simulink model "dSpaceModel_2"  (R2023a)
settings: Solver=ode1  StartTime=0.0  StopTime=inf  FixedStep=0.001  RelTol=1e-3
PostLoadFcn:
  | , if any(exist('dsrtsu_mdlpostloadfcn', 'file') ~= 0), dsrtsu_mdlpostloadfcn('Execute', bdroot); end,
InitFcn:
  | , if any(exist('rtifpga_mdlclblib', 'file') ~= 0), rtifpga_mdlclblib('Init', bdroot); end,
model workspace (MAT data in the model file):
  mode = 2
libraries: rti1202serlib x5, simulink x2, svdutilitieslib x1
(part 3 of 3)

== stateflow chart dSpaceModel_2/RS485/THERMO FSM ==
  state IDLE [commented out]
    during:
    req_valid=false;
    if after(100, msec)
    req_valid=true;
    end
  state WAIT [commented out]
    entry:
    req_valid=false;
  state INIT
    % ZKDM replies are FC profile, fixed 8 bytes with BCC (XOR)
    str = "A005";
    addr = uint8('A005');
    expect_addr      = addr;      % uint8 (the on-wire address byte you use)
    expect_addr_len    = strlength(str);
    expect_len       = uint8(0);
    expect_crc_kind      = uint8(0);     % 0 = BCC/XOR
    % parser outputs (safe defaults)
    temp_rel    = 0.0;
    % Request interface defaults
    req_valid   = false;
    req_len     = uint8(0);
    %device
    last_ok_ms = uint32(0);
    comm_err_count = uint16(0);
  state READY
    entry:
    req_valid= false;
    READY_to_WAIT_GRANT = false;
    during:
    % Pacing: only build/send if enough time passed since last OK or last try
    if after(min_period_ms, msec)
    % Build the telegram NOW from live inputs
    [tx_buf, tx_len]  =  thermCom1(commandType, setpoint);
    %debug_pcd2 = tx_buf(1, 6:7);
    %debug_command = debug_cmnd(setpoint);
    % Advertise request to BUS MASTER
    req_bytes = tx_buf;
    req_len = tx_len;
    expect_addr  = addr;
    expect_len   = uint8(0);
    expect_crc_kind = uint8(0); % BCC XOR
    req_valid    = true;
    % move to wait for arbitration
    READY_to_WAIT_GRANT = true;
    end
  state COOLDOWN
    %nothing; the 'after(min_period_ms,msec)' in READY controls rate
  state HANDLE_ERR
    entry:
    comm_err_count = comm_err_count + 1;
    % Optionally: set FU_bereit=false when repeated timeouts
  state PARSE
    entry:
    temp_rel= parse_thermo_reply1(resp_data(1:64));
    % Master should have validated addr/len/BCC already; still allow a local guard:
    %if (bcc_ok)
    %tic();
    %last_ok_ms = uint32(toc());  % or leave; master’s timing is enough
    %else
    %comm_err_count = comm_err_count + uint16(1);
    %end
  state WAIT_RESP
    during:
    % keep req_valid_ZKDM = false to avoid re-queuing while current tx is active
    req_valid = false;
  state WAIT_GRANT
    %hold req_valid_ZKDM high until master grants
    entry:
    READY_to_WAIT_GRANT = false;
  (default) -> IDLE [commented out]
  WAIT -> IDLE [commented out] : [resp_ok || resp_err]
  IDLE -> WAIT [commented out] : [(after(1,tick))]
  (default) -> INIT
  COOLDOWN -> READY : [after(1,tick)]
  INIT -> READY : [(after(1,tick))]
  HANDLE_ERR -> COOLDOWN : [(after(1,tick))]
  PARSE -> COOLDOWN : after(min_period_ms,msec)
  WAIT_RESP -> HANDLE_ERR [order 2] : [resp_err>0]
  WAIT_GRANT -> HANDLE_ERR [order 2] : [resp_err>0]
  READY -> WAIT_GRANT : [    READY_to_WAIT_GRANT == true]
  WAIT_GRANT -> WAIT_RESP [order 1] : [grant==true]
  WAIT_RESP -> PARSE [order 1] : [resp_ok==true]
  data: address function_input; addressLength function_input; commandType function_input; setpoint function_input; setpointReduced function_input; setpointReducedLength function_input; command function_output; numBytes function_output; ctl_invalid function_input; run_en function_input; ref_pct function_input; bytes function_output; n function_output; commandType function_input; setpoint function_input; command function_output; length function_output; q14 function_input; pct function_output; commandType function_input; setpoint function_input; command function_output; outLen function_output; cfg function_output; buf function_input; n function_input; cfg function_input; ok function_output; status_word function_output uint16 size=1; freq_percent function_output; u function_input; y function_output; invalid_control_word function_input; active function_input; setpoint function_input; command function_output; off_set function_input; u function_input uint8 size=[1 64]; PCD1_1 function_output uint8 size=1; PCD1_2 function_output uint8 size=1; freq_rel_percent function_output double size=1; status_word function_output uint16 size=1; fu_ctrl_ready function_output boolean size=1; fu_ready function_output boolean size=1; fault_trip function_output boolean size=1; fault_no_trip function_output boolean size=1; bus_control_active function_output boolean size=1; bcc_ok function_output boolean size=1; setpoint function_input; cmnds function_output; pcd2 function_input; mode function_input; out function_output; b_in function_input; REV8 function_input; mode function_input; y function_output; REV8 function_output; active input boolean size=1; setpoint input double size=1; req_valid output boolean size=1; req_bytes output uint8 size=[1 127]; req_len output uint8 size=1; expect_addr output uint8; grant input boolean size=1; resp_ok input boolean size=1; resp_err input uint8 size=1; resp_data input uint8 size=[1 127]; resp_len input uint8 size=1; expect_len output uint8 size=1; expect_crc_kind output uint8 size=1; addr local uint8; invalid_flag local boolean size=1 =false; min_period_ms local uint8 size=1 =50; off_set local double size=1 =0; tx_len local uint8 size=1 =0; PCD1_1 local uint8 size=1; PCD1_2 local uint8 size=1; bus_ctrl_active local boolean size=1 =true; debug_command local uint16 size=[1 8]; debug_pcd2 local uint8 size=[1 2]; fault_no_trip local boolean size=1; fault_trip local boolean size=1; temp_rel local double size=1; fu_ctrl_ready local boolean size=1; fu_ready local boolean size=1; last_ok_ms local uint32 size=1; status_word local uint16 size=1; READY_to_WAIT_GRANT local; bcc_ok local boolean size=1; comm_err_count local uint16 size=1; tx_buf local uint8 size=[1 127]; commandType input uint8 size=1; str local string; expect_addr_len local double size=1
  function [command, numBytes] = thermoCommand(address, addressLength, commandType, setpoint, setpointReduced, setpointReducedLength):
    | function [command, numBytes] = thermoCommand(address, addressLength, commandType, setpoint, setpointReduced, setpointReducedLength)
    | 
    | % Initialize the command array and number of bytes
    | command  = zeros(1, 127, 'uint8');
    | numBytes = uint8(0);
    | 
    | % Insert the thermostat address into the command array
    | indexStart = 1;
    | indexEnd   = addressLength;
    | command(indexStart:indexEnd) = address(1:addressLength);
    | 
    | % Determine the command vector based on the provided command type (commandType)
    | switch commandType
    |     case 0
    |         commandVector = uint8('out_mode_05');  % Stop the thermostat
    |     case 1
    |         commandVector = uint8('out_sp_00');    % Set working temperature 'T'
    |     case 2
    |         commandVector = uint8('in_pv_00');     % Actual bath temperature
    |     case 3
    |         commandVector = uint8('in_pv_01');     % Current heat output (%)
    |     case 4
    |         commandVector = uint8('status');       % Status and error messages
    |     otherwise
    |         error('Invalid command: commandType must be in [0, 4].');
    | end
    | 
    | % Insert the command vector into the command array
    | commandLength = length(commandVector);
    | indexStart = indexEnd + 1;
    | indexEnd   = indexStart + commandLength - 1;
    | 
    | % Check for potential overflow
    | if indexEnd > length(command)
    |     error('Command array overflow: cannot add command.');
    | end
    | command(indexStart:indexEnd) = commandVector(1:commandLength);
    | 
    | % If `setpoint` is not NaN, append it to the command
    | if ~isnan(setpoint)
    |     % Insert a space (ASCII 32) between the command and the `setpoint`
    |     indexStart = indexEnd + 1;
    |     command(indexStart) = uint8(32); % Space character
    |     indexEnd = indexStart; % Update indexEnd to the newly added space
    | 
    |     % Depending on `commandType`, handle setpoint insertion differently
    |     if commandType == 0
    |         % For command type 0, transform setpoint to character
    |         command(indexEnd + 1) = uint8(setpoint + 48); % Convert number to corresponding ASCII character
    |         indexEnd = indexEnd + 1; % Move to the next index
    |     else
    |         % For other commands, use `setpointReduced`
    |         indexStart = indexEnd + 1;
    |         indexEnd   = indexStart + setpointReducedLength - 1;
    | 
    |         % Check for potential overflow
    |         if indexEnd > length(command)
    |             error('Command array overflow: cannot add setpointReduced.');
    |         end
    |         command(indexStart:indexEnd) = setpointReduced(1:setpointReducedLength);
    |     end
    | end
    | 
    | % Insert the end character (Carriage Return)
    | indexStart = indexEnd + 1;
    | command(indexStart) = uint8(13); % ASCII for Carriage Return
    | 
    | % Update numBytes to the total number of valid bytes filled in the command
    | numBytes = uint8(indexStart);
    | 
    | end
  function [bytes, n] = build_pcd8(ctl_invalid, run_en, ref_pct):
    | function [bytes, n] = build_pcd8(ctl_invalid, run_en, ref_pct)
    |     % Call your tested MATLAB Function (Create FC-Protocol Command 8-Bytes)
    |     % Or inline the builder. Must return [1x8 uint8] and n=8.
    |     n = unit8(8);
    |     [bytes, n] = FC_Command_8Bytes(ctl_invalid, run_en, ref_pct);
    | end
  function [command, length] = thermCom (commandType, setpoint):
    | function [command, length] = thermCom (commandType, setpoint)
    |     strr = 'A005';
    |     address = uint8(strr);
    |     addressLength = strlength(strr);
    |     tmp = sprintf('%.2f', setpoint);
    |     setpointReduced = uint8(tmp);
    |     setpointReducedLength = strlength(tmp);
    |     [command, length] = thermoCommand(address, addressLength, commandType, setpoint, setpointReduced, setpointReducedLength);
    | end
  function pct = q14_to_percent(q14):
    | function pct = q14_to_percent(q14)
    |     pct = 100.0 * double(q14) / 16384.0;
    | end
  function [command, outLen] = thermCom1(commandType, setpoint):
    | function [command, outLen] = thermCom1(commandType, setpoint)
    |     %#codegen
    |     
    |     address = uint8('A005_');
    |     addressLength = uint32(4);
    |     
    |     MAXSP = 16; % enough for "-999999.99"
    |     setpointReduced = zeros(1, MAXSP, 'uint8');
    |     setpointReducedLength = uint32(0);
    |     
    |     % ---- format setpoint to "%.2f" into fixed buffer ----
    |     x = double(setpoint);
    |     if isnan(x) || isinf(x)
    |         % "NaN" fallback
    |         setpointReduced(1:3) = uint8('NaN');
    |         setpointReducedLength = uint32(3);
    |     else
    |         % sign
    |         idx = uint32(1);
    |         if x < 0
    |             setpointReduced(idx) = uint8('-'); idx = idx + 1;
    |             x = -x;
    |         end
    |     
    |         % round to 2 decimals
    |         x100 = floor(x * 100 + 0.5);          % integer of value*100 rounded
    |         ip = floor(x100 / 100);               % integer part
    |         fp = x100 - ip * 100;                 % fractional part 0..99
    |     
    |         % integer part to ASCII (no leading zeros)
    |         % collect digits in reverse then write back
    |         tmpDigits = zeros(1, 10, 'uint8');
    |         dlen = uint32(0);
    |         if ip == 0
    |             dlen = uint32(1);
    |             tmpDigits(1) = uint8('0');
    |         else
    |             while ip > 0 && dlen < 10
    |                 dlen = dlen + 1;
    |                 digit = uint8(mod(ip,10));
    |                 tmpDigits(dlen) = uint8('0') + digit;
    |                 ip = floor(ip / 10);
    |             end
    |         end
    |         % write digits reversed
    |         for k = dlen:-1:1
    |             setpointReduced(idx) = tmpDigits(k);
    |             idx = idx + 1;
    |         end
    |     
    |         % decimal point
    |         setpointReduced(idx) = uint8('.'); idx = idx + 1;
    |     
    |         % two fractional digits (always)
    |         tens = uint8(floor(fp / 10));
    |         ones = uint8(fp - double(tens) * 10);
    |         setpointReduced(idx) = uint8('0') + tens; idx = idx + 1;
    |         setpointReduced(idx) = uint8('0') + ones; idx = idx + 1;
    |     
    |         setpointReducedLength = idx - 1;
    |     end
    |     
    |     [command, outLen] = thermoCommand( ...
    |         address, addressLength, commandType, setpoint, ...
    |         setpointReduced, setpointReducedLength);
    | end
  function cfg = zkdm_resp_map:
    | function cfg = zkdm_resp_map()
    | % Positions are 1-based indices in the received byte vector
    | cfg.idx_stx   = 1;
    | cfg.idx_len   = 2;
    | cfg.idx_addr  = 3;
    | cfg.idx_statH = 4;
    | cfg.idx_statL = 5;
    | cfg.idx_freqH = 6;
    | cfg.idx_freqL = 7;
    | cfg.idx_bcc   = 8;
    | 
    | cfg.expect_len = 8;        % total bytes
    | cfg.endian_hi_lo = true;   % Q14 is [HI, LO]
    | cfg.q14_fullscale = 16384; % 100%
    | end
  function [ok, status_word, freq_percent] = parse_fc_status(buf, n, cfg):
    | function [ok, status_word, freq_percent] = parse_fc_status(buf, n, cfg)
    | % buf: uint8 vector of the validated reply
    | % n  : actual length (== cfg.expect_len if master validated length)
    | % cfg: map from zkdm_resp_map()
    | 
    | ok = false;
    | status_word = uint16(0);
    | freq_percent = 0.0;
    | 
    | % Basic shape check (defensive)
    | if n < cfg.expect_len
    |     return;
    | end
    | 
    | % Status word (Bytes 4..5 by default)
    | stat_hi = uint16(buf(cfg.idx_statH));
    | stat_lo = uint16(buf(cfg.idx_statL));
    | status_word = bitor( stat_lo, bitshift(stat_hi, 8) );  % (HI,LO) → 16-bit
    | 
    | % Q14 output frequency (Bytes 6..7 by default)
    | bH = uint16(buf(cfg.idx_freqH));
    | bL = uint16(buf(cfg.idx_freqL));
    | if cfg.endian_hi_lo
    |     q14 = bitor( bL, bitshift(bH, 8) );     % HI,LO on the wire → H<<8 | L
    | else
    |     q14 = bitor( bH, bitshift(bL, 8) );     % LO,HI variant if needed
    | end
    | 
    | % Clip and scale to percent
    | if q14 > cfg.q14_fullscale
    |     q14 = cfg.q14_fullscale;   % sanity
    | end
    | freq_percent = 100.0 * double(q14) / double(cfg.q14_fullscale);
    | 
    | ok = true;
    | end
  function y = parse_thermo_reply1(u):
    | function y = parse_thermo_reply1(u)
    |     %#codegen
    |     % u: uint8 vector (e.g., 1x64)
    |     % returns y as double (NaN if invalid)
    |     
    |     y = NaN;
    |     
    |     N = int32(numel(u));
    |     if N == 0
    |         return;
    |     end
    |     
    |     CR = uint8(13);
    |     US = uint8('_');
    |     
    |     % ---------- find end (before CR) ----------
    |     endIdx = N;
    |     for i = int32(1):N
    |         if u(i) == CR
    |             endIdx = i - 1;
    |             break;
    |         end
    |     end
    |     if endIdx < 1
    |         return;
    |     end
    |     
    |     % ---------- find first underscore ----------
    |     sepIdx = int32(0);
    |     for i = int32(1):endIdx
    |         if u(i) == US
    |             sepIdx = i;
    |             break;
    |         end
    |     end
    |     if sepIdx == 0 || sepIdx == endIdx
    |         return;
    |     end
    |     
    |     % ---------- parse number after underscore ----------
    |     i = sepIdx + 1;
    |     
    |     % % skip spaces (optional)
    |     % while i <= endIdx && u(i) == uint8(32)
    |     %     i = i + 1;
    |     % end
    |     % if i > endIdx
    |     %     return;
    |     % end
    |     
    |     % sign
    |     sgn = 1.0;
    |     if u(i) == uint8('-')
    |         sgn = -1.0;
    |         i = i + 1;
    |     elseif u(i) == uint8('+')
    |         i = i + 1;
    |     end
    |     if i > endIdx
    |         return;
    |     end
    |     
    |     % integer part
    |     val = 0.0;
    |     hasDigit = false;
    |     while i <= endIdx
    |         c = u(i);
    |         if c >= uint8('0') && c <= uint8('9')
    |             val = val * 10.0 + double(c - uint8('0'));
    |             hasDigit = true;
    |             i = i + 1;
    |         else
    |             break;
    |         end
    |     end
    |     
    |     % fractional part
    |     if i <= endIdx && u(i) == uint8('.')
    |         i = i + 1;
    |         place = 0.1;
    |         while i <= endIdx
    |             c = u(i);
    |             if c >= uint8('0') && c <= uint8('9')
    |                 val = val + double(c - uint8('0')) * place;
    |                 place = place * 0.1;
    |                 hasDigit = true;
    |                 i = i + 1;
    |             else
    |                 break;
    |             end
    |         end
    |     end
    |     
    |     if ~hasDigit
    |         return;
    |     end
    |     
    |     y = sgn * val;
    | end
  function command = fcn(invalid_control_word, active, setpoint, off_set):
    | % Generates a telegram of the FC protocol for communication with a Danfoss frequency converter,
    | % telegram type: Process block (PCD) – 4 bytes
    | %
    | %##################################################################################
    | %Danfoss control word according to FC profile
    | %----------------------------------------------------------------------------------
    | %| Bit|                        Bit value = 0 |                     Bit value = 1  |
    | %|----|--------------------------------------|------------------------------------|
    | %| 00 | selection between the four "3-10 Preset reference [0]...[3]"             |
    | %| 01 | --""--                                                                   |
    | %|----|--------------------------------------|------------------------------------|
    | %| 02 |             DC brake and stop        |             performs ramp          |
    | %|----|--------------------------------------|------------------------------------|
    | %| 03 | lets the motor coast                 | starts the motor if conditions are met |
    | %|----|--------------------------------------|------------------------------------|
    | %| 04 | motor speed decreases until stop     |                                    |
    | %|----|--------------------------------------|------------------------------------|
    | %| 05 | current output frequency is stored   |                                    |
    | %|----|--------------------------------------|------------------------------------|
    | %| 06 | stop using ramp time                 | starts the motor if conditions are met |
    | %|----|--------------------------------------|------------------------------------|
    | %| 07 | no reset                             | reset                              |
    | %|----|--------------------------------------|------------------------------------|
    | %| 08 |                                      | output frequency "3-19 Jog [RPM]"  |
    | %|----|--------------------------------------|------------------------------------|
    | %| 09 | ramp 1 active ("3-41" and "3-42")    | ramp 2 active ("3-51" and "3-52")  |
    | %|----|--------------------------------------|------------------------------------|
    | %| 10 | control word is ignored              | control word is used               |
    | %|----|--------------------------------------|------------------------------------|
    | %| 11 | relay 01 not activated               | relay 01 activated                 |
    | %|----|--------------------------------------|------------------------------------|
    | %| 12 | relay 04 not activated               | relay 04 activated                 |
    | %|----|--------------------------------------|------------------------------------|
    | %| 13 | parameter set selection "0-10" and "8-55"                                |
    | %| 14 |                                                                            |
    | %|----|--------------------------------------|------------------------------------|
    | %| 15 | no reversal                          | reversal                           |
    | %----------------------------------------------------------------------------------
    | %##################################################################################
    | 
    | function command = fcn(invalid_control_word, active, setpoint, off_set)
    | 
    | if setpoint < 0
    |         error('setpoint must be non-negative.');
    | end
    | 
    | command = zeros(1, 127, 'uint8');
    | startzeichen = uint8(2);    % Start character (STX)
    | telegrammlaenge = uint8(6); % Specifies telegram length: 6 or 14 data bytes (data bytes + address byte + checksum)
    | adresse = 0b01111101;       % Address 125 in binary, address of the frequency converter (FU)
    |                             % Address format 1–126 => Bit 7 = 1; FU address “10” => Bit 0–6
    | pcd1_1 = 0b00000100;        % Control word (CTW) bits 15 to 08
    | pcd1_2 = 0b00100100;        % Control word (CTW) bits 07 to 00 ... before change: 0b00101110;
    | bcc = 0;                    % Data control byte, Block Check Character (BCC)
    | 
    | % modify the flag
    | if (invalid_control_word == false)
    |     pcd1_1 = bitor(pcd1_1, 0b00100000); 
    |     % If invalid_flag is `false`, the result will change `pcd11` to `0b00100000`, indicating that the control word is now in use.
    | end
    | 
    | if (active == true)
    |     pcd1_2 = bitor(pcd1_2, 0b01111100); % set 02, 03, 04, 05, 06 to 1
    |     pcd1_1 = bitor(pcd1_1, 0b00000100); % Starts the motor; "0": the frequency converter lets the motor coast
    | end
    | 
    | %%- `command(4) = pcd1_1;`
    |   % - Value: This byte is constructed based on the input conditions (`steuerwort_invalid` and `aktiv`).
    |   % - It starts with `0b00000000` (initial value) and may have bits set:
    |   %   - Bit 5 is set to 1 if `steuerwort_invalid` is false (valid control word).
    |   %   - Bit 4 is set to 1 if `aktiv` is true (start command).
    |   % - As a result, if `aktiv` is true, the value changes:
    |   %     - From: `0b00100000`
    |   %     - To:   `0b00110000` (decimal 48), indicating that the motor should start.
    | 
    | % scale the speed setpoint
    | % Example: convert 50% speed to 16-bit integer
    | % 50% = (16384 / 100 * 50) = 8192
    | % 8192 = 0b1000000000000000 (binary)
    | 
    | if (setpoint <= off_set)
    |     setpoint = 0;
    | else
    |     setpoint = setpoint - off_set;
    | end
    | 
    | soll = setpoint * (16384 / 100); 
    | pcd2 = typecast(int16(soll),'uint8');
    | % pcd2 = flip(pcd2);
    | 
    | %This is a 16-bit integer converted to two bytes that represents the desired speed (drehzahl_Sollwert) scaled to a proper range.
    |    %- The speed is scaled by multiplying the `drehzahl_Sollwert` by `(16384 / 100)`, allowing for a representation of the speed setting as a 16-bit integer.
    |    %- This is then converted from an `int16` to `uint8`, giving two bytes: `pcd2(1)` and `pcd2(2)`, with the bytes being flipped to match byte order expectations.
    | 
    | bcc = bitxor(startzeichen, telegrammlaenge);
    | bcc = bitxor(bcc, adresse);
    | bcc = bitxor(bcc, pcd1_1);
    | bcc = bitxor(bcc, pcd1_2);
    | bcc = bitxor(bcc, pcd2(1));
    | bcc = bitxor(bcc, pcd2(2));
    | 
    | command(1) = startzeichen;
    | command(2) = telegrammlaenge;
    | command(3) = adresse;
    | command(4) = pcd1_1; %This byte functions as part of the control command to the motor, determining how it should behave.
    | command(5) = pcd1_2; %This byte also forms part of the control command. It usually contains predefined flags or control commands as per the motor's specification.
    | command(6:7) = pcd2; %This part of the command specifies the desired speed for the motor. from the user sollwert.
    | command(8) = bcc;
    | 
    | %example message:
    | 
    | %Address: 118 Motor Activation Flag: True Target Speed: 89% BCC is valid
    | %2 6 118 48 46 56 246 162
  function [PCD1_1, PCD1_2, freq_rel_percent, ...:
    | function [PCD1_1, PCD1_2, freq_rel_percent, ...
    |           status_word, ...
    |           fu_ctrl_ready, fu_ready, fault_trip, fault_no_trip, bus_control_active, ...
    |           bcc_ok] = parse_fc_reply(u)
    | %#codegen
    | % Parse 8-byte FC reply built by your current build_fc_rx_telegram()
    | % Layout: [STX, LEN, ADDR, STW_HI, STW_LO, OUT_HI, OUT_LO, BCC]
    | % Bit mapping (matches your TX builder with msbpos()):
    | %   fu_ctrl_ready      -> bit15
    | %   fu_ready           -> bit14
    | %   fault_trip         -> bit13
    | %   fault_no_trip      -> bit12
    | %   bus_control_active -> bit6
    | 
    |     % ---- basic checks ----
    |     if numel(u) < 8
    |         error('parse_fc_reply:BadLength','u must have at least 8 bytes');
    |     end
    |     u = uint8(u(:).'); % row uint8
    | 
    |     % ---- BCC (XOR of bytes 1..7) ----
    |     b = uint8(0);
    |     for k = 1:7
    |         b = bitxor(b, u(k));
    |     end
    |     bcc_ok = (b == u(8));
    | 
    |     % ---- status word bytes ----
    |     PCD1_1 = u(4); % high byte (bits 15..8)
    |     PCD1_2 = u(5); % low  byte (bits 7..0)
    | 
    |     % Full 16-bit status word: [HI<<8 | LO]
    |     status_word = bitor( bitshift(uint16(PCD1_1),8), uint16(PCD1_2) );
    | 
    |     % Helper to read a single LSB-indexed bit (0..15)
    |     getbit = @(w, n) bitand(w, bitshift(uint16(1), n)) ~= 0;
    | 
    |     % ---- flags (LSB indexing) matching your TX mapping ----
    |     fu_ctrl_ready      = getbit(status_word, 15); % msbpos(0)
    |     fu_ready           = getbit(status_word, 14); % msbpos(1)
    |     fault_trip         = getbit(status_word, 13); % msbpos(2)
    |     fault_no_trip      = getbit(status_word, 12); % msbpos(3)
    |     bus_control_active = getbit(status_word,  6); % msbpos(9)
    | 
    |     % ---- OUT (Q14) -> relative frequency (%) ----
    |     q14 = bitor( bitshift(uint16(u(6)),8), uint16(u(7)) );
    |     freq_rel_percent = double(q14) * (100.0/16384.0);
    | end
  function cmnds = debug_cmnd(setpoint):
    | function cmnds = debug_cmnd(setpoint)
    |     
    |     if setpoint < 0
    |             error('setpoint must be non-negative.');
    |     end
    |     
    |     command = zeros(1, 8, 'uint16');
    |     soll = setpoint * (16384 / 100); 
    |     pcd2 = uint16(round(soll));
    |     all = pcd2_flipcases(pcd2);
    |     cmnds = all.values;
    | end
  function out = pcd2_flipcases(pcd2, mode):
    | function out = pcd2_flipcases(pcd2, mode)
    | % Modes (YOUR numbering):
    | %   0: I
    | %   1: N
    | %   2: R    (per-byte bit reverse)
    | %   3: B    (byte swap)
    | %   4: BR   (byte swap + per-byte bit reverse)
    | %   5: NR
    | %   6: NB
    | %   7: NBR
    | 
    |     x = uint16(pcd2);
    |     origSize = size(x);
    |     x = x(:);
    | 
    |     b = reshape(typecast(x, 'uint8'), 2, []).';  % N-by-2 uint8, [LSB MSB]
    | 
    |     persistent REV8
    |     if isempty(REV8)
    |         REV8 = make_rev8_lut();
    |     end
    | 
    |     % Internal bitmask encoding (N=1, B=2, R=4) is convenient,
    |     % but you want a different external mode order:
    |     % external_mode -> internal_mask
    |     map = uint8([0 1 4 2 6 5 3 7]);
    | 
    |     labels = {"I","N","R","B","BR","NR","NB","NBR"};
    | 
    |     if nargin < 2 || isempty(mode)
    |         vals = zeros(numel(x), 8, 'uint16');
    |         for m = 0:7
    |             vals(:, m+1) = apply_mode(b, REV8, map(m+1));
    |         end
    |         out = struct();
    |         out.modes  = uint8(0:7);
    |         out.labels = labels;
    |         out.values = vals;                          % (numel(x) x 8)
    |         out.asArray = reshape(vals, [origSize, 8]); % append dim=8
    |         return;
    |     end
    | 
    |     mode = uint8(mode);
    |     if any(mode > 7)
    |         error("mode must be an integer in 0..7.");
    |     end
    | 
    |     if isscalar(mode)
    |         y = apply_mode(b, REV8, map(mode+1));
    |         out = reshape(y, origSize);
    |         return;
    |     end
    | 
    |     mode = mode(:).';
    |     vals = zeros(numel(x), numel(mode), 'uint16');
    |     for k = 1:numel(mode)
    |         vals(:, k) = apply_mode(b, REV8, map(mode(k)+1));
    |     end
    |     out = reshape(vals, [origSize, numel(mode)]);
    | end
  function y = apply_mode(b_in, REV8, mode):
    | function y = apply_mode(b_in, REV8, mode)
    |     % b_in: N-by-2 uint8, [LSB MSB]
    |     b = b_in;
    | 
    |     doN = bitand(mode, 1) ~= 0;
    |     doB = bitand(mode, 2) ~= 0;
    |     doR = bitand(mode, 4) ~= 0;
    | 
    |     if doN
    |         b = bitcmp(b);
    |     end
    | 
    |     if doR
    |         % per-byte bit reverse via LUT
    |         b = REV8(double(b) + 1);
    |     end
    | 
    |     if doB
    |         b = b(:, [2 1]); % swap bytes
    |     end
    | 
    |     % Back to uint16 (bytes must be laid out as [LSB MSB] for typecast)
    |     bb = b.';                        % 2-by-N
    |     y  = typecast(bb(:), 'uint16');  % N-by-1 uint16
    | end
  function REV8 = make_rev8_lut:
    | 
    | % function LUT = make_rev8_lut()
    | %     % Pure bit-ops LUT: LUT(v+1) = bit-reverse of uint8(v)
    | %     LUT = zeros(256, 1, 'uint8');
    | %     for v = 0:255
    | %         x = uint8(v);
    | %         r = uint8(0);
    | %         % reverse 8 bits
    | %         for k = 0:7
    | %             r = bitor(r, bitshift(bitand(x, bitshift(uint8(1), k)), 7-k) ~= 0);
    | %         end
    | %         LUT(v+1) = r;
    | %     end
    | % end
    | 
    | function REV8 = make_rev8_lut()
    |     %REV8(i) = bit-reversal of uint8(i-1)
    |     
    |     x = uint8(0:255);
    |     REV8 = zeros(1,256,'uint8');
    |     
    |     for i = 1:256
    |         b = x(i);
    |         r = uint8(0);
    |         for k = 0:7
    |             % bitget returns double -> cast to uint8 before shifting
    |             r = bitor(r, bitshift(uint8(bitget(b, k+1)), 7-k));
    |         end
    |         REV8(i) = r;
    |     end
    | end

== matlab function dSpaceModel_2/RS485/MATLAB Function2 ==
  data: u input; PCD1_1 output; PCD1_2 output; freq_rel_percent output; status_word output; fu_ctrl_ready output; fu_ready output; fault_trip output; fault_no_trip output; bus_control_active output; bcc_ok output
function [PCD1_1, PCD1_2, freq_rel_percent, ...
          status_word, ...
          fu_ctrl_ready, fu_ready, fault_trip, fault_no_trip, bus_control_active, ...
          bcc_ok] = parse_fc_reply(u)
%#codegen
% Parse 8-byte FC reply built by your current build_fc_rx_telegram()
% Layout: [STX, LEN, ADDR, STW_HI, STW_LO, OUT_HI, OUT_LO, BCC]
% Bit mapping (matches your TX builder with msbpos()):
%   fu_ctrl_ready      -> bit15
%   fu_ready           -> bit14
%   fault_trip         -> bit13
%   fault_no_trip      -> bit12
%   bus_control_active -> bit6

    % ---- basic checks ----
    if numel(u) < 8
        error('parse_fc_reply:BadLength','u must have at least 8 bytes');
    end
    u = uint8(u(:).'); % row uint8

    % ---- BCC (XOR of bytes 1..7) ----
    b = uint8(0);
    for k = 1:7
        b = bitxor(b, u(k));
    end
    bcc_ok = (b == u(8));

    % ---- status word bytes ----
    PCD1_1 = u(4); % high byte (bits 15..8)
    PCD1_2 = u(5); % low  byte (bits 7..0)

    % Full 16-bit status word: [HI<<8 | LO]
    status_word = bitor( bitshift(uint16(PCD1_1),8), uint16(PCD1_2) );

    % Helper to read a single LSB-indexed bit (0..15)
    getbit = @(w, n) bitand(w, bitshift(uint16(1), n)) ~= 0;

    % ---- flags (LSB indexing) matching your TX mapping ----
    fu_ctrl_ready      = getbit(status_word, 15); % msbpos(0)
    fu_ready           = getbit(status_word, 14); % msbpos(1)
    fault_trip         = getbit(status_word, 13); % msbpos(2)
    fault_no_trip      = getbit(status_word, 12); % msbpos(3)
    bus_control_active = getbit(status_word,  6); % msbpos(9)

    % ---- OUT (Q14) -> relative frequency (%) ----
    q14 = bitor( bitshift(uint16(u(6)),8), uint16(u(7)) );
    freq_rel_percent = double(q14) * (100.0/16384.0);
end

== matlab function dSpaceModel_2/RS485/Subsystem2/MATLAB Function ==
  data: u input; PCD1_1 output; PCD1_2 output; PCD2 output
function [PCD1_1, PCD1_2, PCD2] = fcn(u)
%Steuerwort
PCD1_1 = u(4);
PCD1_2 = u(5);

%berechnet aktuelle Ausgangsfrequenz als relativen Wert in Prozent
PCD2 = (u(6)*256 + u(7)) * (100 / 16384);

== matlab function dSpaceModel_2/RS485/MATLAB Function3 ==
  data: fu_ctrl_ready input; u output; fu_ready input; fault_trip input; fault_no_trip input; bus_control_active input; freq_rel_percent input; addr input
function u = build_fc_rx_telegram(fu_ctrl_ready, fu_ready, fault_trip, fault_no_trip, bus_control_active, freq_rel_percent, addr)
%#codegen
% Build an 8-byte Danfoss FC "reply" telegram:
%   [STX, LEN, ADDR, STW_HI, STW_LO, OUT_HI, OUT_LO, BCC]
%
% Inputs:
%   fu_ctrl_ready       : logical  % maps to STW bit 0
%   fu_ready            : logical  % maps to STW bit 1
%   fault_trip          : logical  % maps to STW bit 2 (trip = hard fault)
%   fault_no_trip       : logical  % maps to STW bit 3 (warning)
%   bus_control_active  : logical  % maps to STW bit 12
%   freq_rel_percent    : double   % 0..100 (%) — will be clamped & rounded to Q14
%   addr                : uint8    % (optional) on-wire FC address byte; default 253
%
% Output:
%   u (1x8 uint8) = FC reply frame you can feed into your parser
%
% Notes:
% - Mapping follows the demo you showed:
%     bit0 = fu_ctrl_ready
%     bit1 = fu_ready
%     bit2 = fault_trip
%     bit3 = fault_no_trip
%     bit12 = bus_control_active
% - OUT is Q14: 0..16384 ↔ 0..100%

    if nargin < 7
        addr = uint8(253);   % default FC on-wire address (e.g., node 125)
    else
        addr = uint8(addr);
    end

    % helper: convert MSB index k (15..0) to bitset() position (1..16)
    msbpos = @(k) 16 - k;
    
    sw = uint16(0);
    if fu_ctrl_ready,      sw = bitset(sw, msbpos(0),  true); end   % bit0
    if fu_ready,           sw = bitset(sw, msbpos(1),  true); end   % bit1
    if fault_trip,         sw = bitset(sw, msbpos(2),  true); end   % bit2
    if fault_no_trip,      sw = bitset(sw, msbpos(3),  true); end   % bit3
    if bus_control_active, sw = bitset(sw, msbpos(9),  true); end   % bit9

    STW_HI = uint8(bitshift(sw, -8));
    STW_LO = uint8(bitand(sw, 255));

    % ---------- OUT (Q14) from percent ----------
    if ~isfinite(freq_rel_percent), freq_rel_percent = 0; end
    freq_rel_percent = max(0, min(100, freq_rel_percent));
    q14 = uint16(round(freq_rel_percent * (16384/100)));
    OUT_HI = uint8(bitshift(q14, -8));
    OUT_LO = uint8(bitand(q14, 255));

    % ---------- assemble frame ----------
    STX = uint8(2);
    LEN = uint8(6);   % addr + 4 data bytes + BCC

    u = zeros(1,8,'uint8');
    u(1) = STX;
    u(2) = LEN;
    u(3) = addr;
    u(4) = STW_HI;
    u(5) = STW_LO;
    u(6) = OUT_HI;
    u(7) = OUT_LO;

    % ---------- BCC (XOR of bytes 1..7) ----------
    bcc = uint8(0);
    for k = 1:7
        bcc = bitxor(bcc, u(k));
    end
    u(8) = bcc;
end
